simulink model "Transformation_V12"  (R2018a)
settings: Solver=FixedStepDiscrete  StartTime=0.0  StopTime=10.0  RelTol=1e-3
InitFcn:
  | Ts_xadc = 0.1;
values from neighbouring files (symbols this model uses):
  T_25MHz = 1/f_25MHz    (= 4e-08)    [TransformationSkript.m]
  T_mech = 2e-08    [TransformationSkript.m]
libraries: hdlsllib x14, simulink x13, simulink_need_slupdate x1
(part 1 of 3)
settings Model: DataTypeOverride=Off  Creator=trichte  LastModifiedBy=Wendel
settings DataIOCC: LimitDataPoints=on  SaveFormat=Array  SaveOutput=off  SaveTime=off
settings OptimizationCC: BlockReduction=off  ConditionallyExecuteInputs=off  DefaultParameterBehavior=Inlined  LifeSpan=inf
settings DebuggingCC: AlgebraicLoopMsg=error  SolverPrmCheckMsg=warning  SingleTaskRateTransMsg=error  AllowSymbolicDim=off  StrictBusMsg=ErrorOnBusTreatedAsVector  SFUnexpectedBacktrackingDiag=warning  SFNoUnconditionalDefaultTransitionDiag=warning  SFExecutionAtInitializationDiag=none
settings HardwareCC: ProdBitPerPointer=32  ProdBitPerSizeT=32  ProdBitPerPtrDiffT=32  ProdLargestAtomicFloat=None  ProdIntDivRoundTo=Undefined  ProdEndianess=Unspecified  ProdWordSize=32  ProdHWDeviceType=ASIC/FPGA->ASIC/FPGA  ProdEqTarget=off
settings ModelReferenceCC: PropagateSignalLabelsOutOfModel=off
settings CodeAppCC: StateflowObjectComments=on
settings GRTTargetCC: TargetLangStandard=C89/C90 (ANSI)  GeneratePreprocessorConditionals=Disable all
settings ConfigComp: CovMetricSettings=dw  CovHtmlReporting=on  CovSaveCumulativeToWorkspaceVar=on  CovSaveSingleToWorkspaceVar=on  CovExternalEMLEnable=off  CovSFcnEnable=off

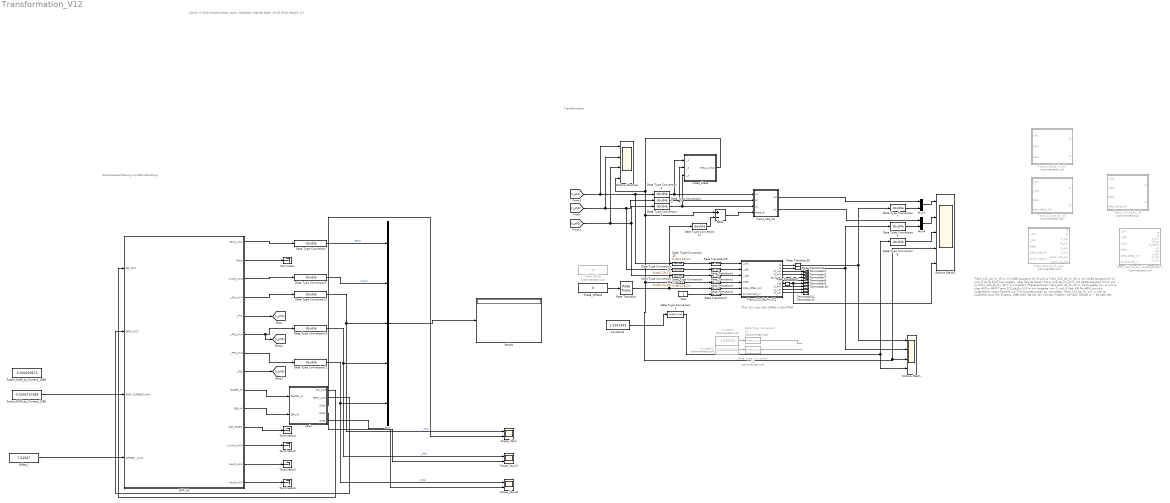
== system Transformation_V12 ==
  note: This V12 runs with 25MHz in the FPGA.
  note: Trans_123_dq_fix_V5 = mit 16Bit Ausgang für id und iq
      | Trans_123_dq_fix_V6 = mit 18 Bit Ausgang für id und iq (iq ist auch hier negativ, aber das ist falsch)
      | Trans_123_dq_fix_V7 = mit 18 Bit Ausgang für id und iq
      | Trans_123_dq_fix_V8 = mit 3 statt 2 Phasenströmen
      | Trans_123_dq_fix_V9 = mit Ausgabe von id und iq über AXI für ARM
      | Trans_123_dq_fix_V10 = mit Ausgabe von i1 und i3 über AXI für ARM und mit zusätzlichem Input-Pipeline um Timingverletzungen zu vermeiden
      | Trans_123_dq_fix_V11 = hier ist zusätzlich auch der Eingang 18Bit breit (da bei der V10 das Problem war das: Sobald iq > 9A geht der Trans-Block nicht mehr richtig...
      | Das liegt an den 16 Bit am Eingang. Sobald ich (wie bei den neunen V11 schon korregiert) 18 Bit am EIngang habe, ist das Problem behoben und der Bereich geht bis bis +/-36 A
      | ...ansonsten is alles wie gehabt. Wegen einheitlichen 18 Bit für alle Größem wird jedoch 18 Bit genutzt!
      | Trans_123_dq_fix_V12 = habe hier nun die dq-Trans von Saidi Said nicht mehr benutzt und bin auf die Verwendung von sinus und cosinus gewechselt.
      | da ich diese bei den VoltageVectors ohnehin benötige. Und hierdurch habe ich auch einen gleichen theta-offset für beide. Außerdem wollte ich alle 3 Ströme nehmen
      | Nach realer Implementierung ist die Genauigkeit von dieser dq-Transformation auch wesentlich genauer (doppelt so gute Bitgenauigkeit)
  note: Stromistwererfassung mit ADC-Wandlung
  note: Transformation
  note: Clarke- & Park-transformation
      |
      | Autor: Sebastian Wendel
      | Date: 26.03.2018
      | Version: 0.1
  Add1 : Sum  Inputs=+-  OutDataTypeStr=Inherit: Same as accumulator
  Constant : Constant  Commented=on  Value=-1.839355
  Constant1 : Constant  Commented=on  Value=0.545410156
  Constant2 : Constant  Value=1.2201433
  DUT_V5 : Subsystem  TreatAsAtomicUnit=on
  Data Type Conversion{,1,3..12} (12 alike) : DataTypeConversion  OutDataTypeStr=double
  Data Type Conversion13 : DataTypeConversion  Commented=on  OutDataTypeStr=fixdt(1,18,11)
  Data Type Conversion14 : DataTypeConversion  Commented=on  OutDataTypeStr=fixdt(1,18,11)
  Data Type Conversion15 : DataTypeConversion  OutDataTypeStr=fixdt(1,18,11)
  Data Type Conversion16 : DataTypeConversion  OutDataTypeStr=fixdt(1,18,11)
  Data Type Conversion17 : DataTypeConversion  OutDataTypeStr=fixdt(1,18,11)
  Data Type Conversion18 : DataTypeConversion  OutDataTypeStr=fixdt(1,24,20)
  Data Type Conversion2 : DataTypeConversion  OutDataTypeStr=fixdt(1,24,20)
  Factor_RAW_to_Current_12Bit : Constant  Value=0.0036747685  OutDataTypeStr=fixdt(0,24,24)
  Factor_RAW_to_Current_16Bit : Constant  Value=0.000229673  OutDataTypeStr=fixdt(0,24,24)
  Mux : Mux  Inputs=5
  Mux3 : Mux  Inputs=2
  Mux4 : Mux  Inputs=2
  Offset_i : Constant  Value=7.52587  OutDataTypeStr=fixdt(0,16,11)
  Rate Transition{,6..7,16} (4 alike) : RateTransition  OutPortSampleTime=T_mech
  Rate Transition{1..5,19} (6 alike) : RateTransition  OutPortSampleTime=T_25MHz
  Scope_Vaux0 : Scope  NumInputPorts=2
  Scope_Vaux8 : Scope  NumInputPorts=2
  Scope_VpVn : Scope  NumInputPorts=2
  Ströme Gleich : Scope  NumInputPorts=4
  Ströme Gleich1 : Scope  NumInputPorts=5
  Ströme Wechsel : Scope  NumInputPorts=4
  Terminator{,1..12} (13 alike) : Terminator
  Test : Constant  OutDataTypeStr=boolean  SampleTime=T_mech
  Theta_Offset : Constant  Commented=on  Value=pi  OutDataTypeStr=fixdt(1,24,20)
  Theta_Offset1 : Constant  Value=0  OutDataTypeStr=fixdt(1,24,20)
  Trans_123_dq : Subsystem
  Trans_123_dq_fix_V11 : Subsystem  Commented=on  TreatAsAtomicUnit=on
  Trans_123_dq_fix_V12 : Subsystem  TreatAsAtomicUnit=on
  Trans_123_dq_fix_V12DoppelteMul : Subsystem  Commented=on  TreatAsAtomicUnit=on
  Trans_123_dq_fix_V3 : Subsystem  Commented=on  TreatAsAtomicUnit=on
  Trans_123_dq_fix_V5 : Subsystem  Commented=on  TreatAsAtomicUnit=on
  Trans_123_dq_fix_V6 : Subsystem  Commented=on  TreatAsAtomicUnit=on
  Values : Display
      settings: Format=hex (Stored Integer)
  meas_theta : Subsystem
  xadc : Subsystem
  wires:
  DUT_V5/1(Temp_AXI4) -> Data Type Conversion/1
  DUT_V5/3(VccInt_AXI4) -> Data Type Conversion1/1
  DUT_V5/4(i_Ph1_AXI4) -> Data Type Conversion3/1
  DUT_V5/7(i_Ph3_AXI4) -> Data Type Conversion11/1
  DUT_V5/6(i_Ph2_AXI4) -> [i_ph2], Data Type Conversion10/1
  Mux/1 -> Values/1
  Data Type Conversion/1 -> Mux/1  "Temp"
  Data Type Conversion3/1 -> Scope_VpVn/1, Mux/3  "i_Ph1"
  Data Type Conversion10/1 -> Scope_Vaux0/1, Mux/4  "i_Ph2"
  Data Type Conversion11/1 -> Scope_Vaux8/1, Mux/5  "i_Ph3"
  Data Type Conversion1/1 -> Mux/2  "VccInt"
  DUT_V5/9(DADDR_IN) -> xadc/1(DADDR_IN)
  DUT_V5/10(DEN_IN) -> xadc/2(DEN_IN)
  xadc/2(DRDY_OUT) -> DUT_V5/2(DRDY_OUT)
  xadc/1(DO_OUT) -> DUT_V5/1(DO_OUT)
  DUT_V5/2(Temp) -> Terminator/1
  DUT_V5/11(ADC_enable) -> Terminator4/1
  Factor_RAW_to_Current_12Bit/1 -> DUT_V5/3(RAW_CURRENT_AXI4)
  Offset_i/1 -> DUT_V5/4(OFFSET_I_AXI4)
  DUT_V5/12(V_VpVn_AXI4) -> Terminator2/1
  DUT_V5/13(Vaux0_AXI4) -> Terminator5/1
  DUT_V5/14(Vaux8_AXI4) -> Terminator6/1
  xadc/3(Sine1) -> Scope_VpVn/2
  xadc/4(Sine2) -> Scope_Vaux0/2
  xadc/5(Sine3) -> Scope_Vaux8/2
  Data Type Conversion2/1 -> Ströme Gleich/4, Data Type Conversion8/1
  Trans_123_dq/1(Ud) -> Mux3/1
  Trans_123_dq/2(Uq) -> Mux4/1
  Mux3/1 -> Ströme Gleich1/1
  Data Type Conversion7/1 -> Mux3/2
  Data Type Conversion6/1 -> Mux4/2
  Mux4/1 -> Ströme Gleich1/2
  Data Type Conversion8/1 -> Ströme Gleich1/3
  meas_theta/1(theta_arctan) -> Ströme Wechsel/4, Ströme Gleich/3, Ströme Gleich1/4, Data Type Conversion18/1, Add1/1
  Data Type Conversion4/1 -> meas_theta/1(I_1), Trans_123_dq/1(L1)
  Data Type Conversion9/1 -> meas_theta/3(I_3), Trans_123_dq/3(L3)
  Data Type Conversion5/1 -> meas_theta/2(I_2), Trans_123_dq/2(L2)
  DUT_V5/5(i_Ph1) -> [i_ph1]
  DUT_V5/8(i_Ph3) -> [i_ph3]
  [i_ph2] -> Ströme Wechsel/2, Data Type Conversion16/1, Data Type Conversion5/1
  Trans_123_dq_fix_V12/1(id) -> Rate Transition16/1
  Trans_123_dq_fix_V12/2(iq) -> Rate Transition6/1
  Data Type Conversion12/1 -> Add1/2
  Add1/1 -> Trans_123_dq/4(theta_el)
  Trans_123_dq_fix_V12/4(iq_AXI) -> Terminator3/1
  Trans_123_dq_fix_V12/3(id_AXI) -> Terminator1/1
  Trans_123_dq_fix_V12/5(dq_Done) -> Terminator7/1
  Trans_123_dq_fix_V12/6(sin) -> Terminator8/1
  [i_ph1] -> Ströme Wechsel/1, Data Type Conversion15/1, Data Type Conversion4/1
  [i_ph3] -> Ströme Wechsel/3, Data Type Conversion17/1, Data Type Conversion9/1
  Data Type Conversion13/1 -> ?
  Data Type Conversion14/1 -> ?
  Rate Transition7/1 -> Ströme Gleich1/5, Terminator9/1
  Test/1 -> Rate Transition5/1
  Trans_123_dq_fix_V12/8(i1_AXI) -> Terminator10/1
  Constant/1 -> Data Type Conversion13/1
  Constant1/1 -> Data Type Conversion14/1
  Constant2/1 -> Data Type Conversion2/1
  Trans_123_dq_fix_V12/9(i2_AXI) -> Terminator11/1
  Trans_123_dq_fix_V12/10(i3_AXI) -> Terminator12/1
  Theta_Offset1/1 -> Rate Transition/1
  Rate Transition19/1 -> Trans_123_dq_fix_V12/1(i_ph1)
  Rate Transition1/1 -> Trans_123_dq_fix_V12/2(i_ph2)
  Rate Transition2/1 -> Trans_123_dq_fix_V12/3(i_ph3)
  Rate Transition3/1 -> Trans_123_dq_fix_V12/4(theta)
  Rate Transition4/1 -> Trans_123_dq_fix_V12/5(theta_offset_AXI)
  Rate Transition5/1 -> Trans_123_dq_fix_V12/6(CurrentValid_in)
  Rate Transition16/1 -> Data Type Conversion7/1, Ströme Gleich/1
  Rate Transition6/1 -> Ströme Gleich/2, Data Type Conversion6/1
  Trans_123_dq_fix_V12/7(cos) -> Rate Transition7/1
  Data Type Conversion15/1 -> Rate Transition19/1
  Data Type Conversion16/1 -> Rate Transition1/1
  Data Type Conversion17/1 -> Rate Transition2/1
  Data Type Conversion18/1 -> Rate Transition3/1
  Rate Transition/1 -> Rate Transition4/1, Data Type Conversion12/1

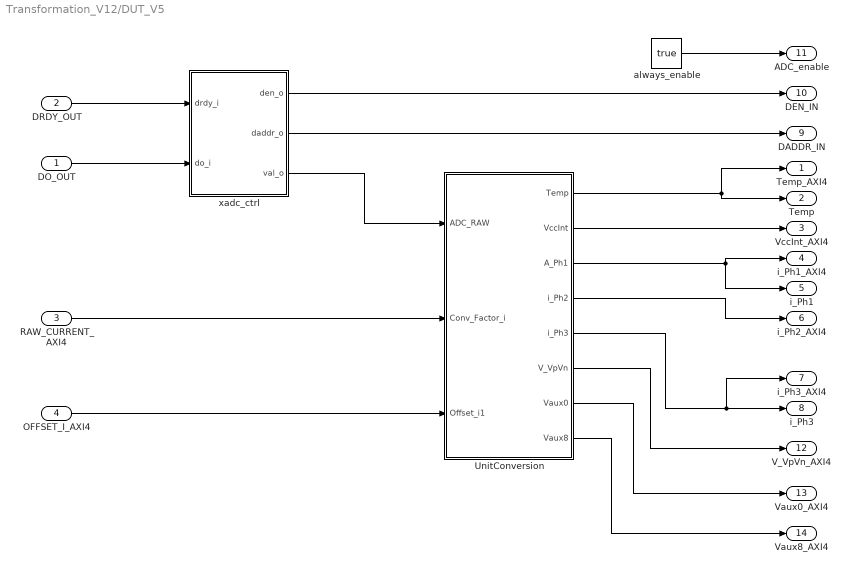
== system Transformation_V12/DUT_V5 ==
  DO_OUT : Inport
  DRDY_OUT : Inport  Port=2
  RAW_CURRENT_AXI4 : Inport  Port=3
  OFFSET_I_AXI4 : Inport  Port=4
  UnitConversion : Subsystem
  always_enable : Constant  Value=true  OutDataTypeStr=boolean
  xadc_ctrl : MATLAB Function  TreatAsAtomicUnit=on
  Temp_AXI4 : Outport
  Temp : Outport  Port=2
  VccInt_AXI4 : Outport  Port=3
  i_Ph1_AXI4 : Outport  Port=4
  i_Ph1 : Outport  Port=5
  i_Ph2_AXI4 : Outport  Port=6
  i_Ph3_AXI4 : Outport  Port=7
  i_Ph3 : Outport  Port=8
  DADDR_IN : Outport  Port=9
  DEN_IN : Outport  Port=10
  ADC_enable : Outport  Port=11
  V_VpVn_AXI4 : Outport  Port=12
  Vaux0_AXI4 : Outport  Port=13
  Vaux8_AXI4 : Outport  Port=14
  wires:
  xadc_ctrl/3(val_o) -> UnitConversion/1(ADC_RAW)
  UnitConversion/5(i_Ph3) -> i_Ph3/1, i_Ph3_AXI4/1
  UnitConversion/3(A_Ph1) -> i_Ph1/1, i_Ph1_AXI4/1
  UnitConversion/4(i_Ph2) -> i_Ph2_AXI4/1
  UnitConversion/2(VccInt) -> VccInt_AXI4/1
  UnitConversion/1(Temp) -> Temp/1, Temp_AXI4/1
  DRDY_OUT/1 -> xadc_ctrl/1(drdy_i)
  DO_OUT/1 -> xadc_ctrl/2(do_i)
  xadc_ctrl/1(den_o) -> DEN_IN/1
  xadc_ctrl/2(daddr_o) -> DADDR_IN/1
  always_enable/1 -> ADC_enable/1
  RAW_CURRENT_AXI4/1 -> UnitConversion/2(Conv_Factor_i)
  UnitConversion/6(V_VpVn) -> V_VpVn_AXI4/1
  OFFSET_I_AXI4/1 -> UnitConversion/3(Offset_i1)
  UnitConversion/7(Vaux0) -> Vaux0_AXI4/1
  UnitConversion/8(Vaux8) -> Vaux8_AXI4/1

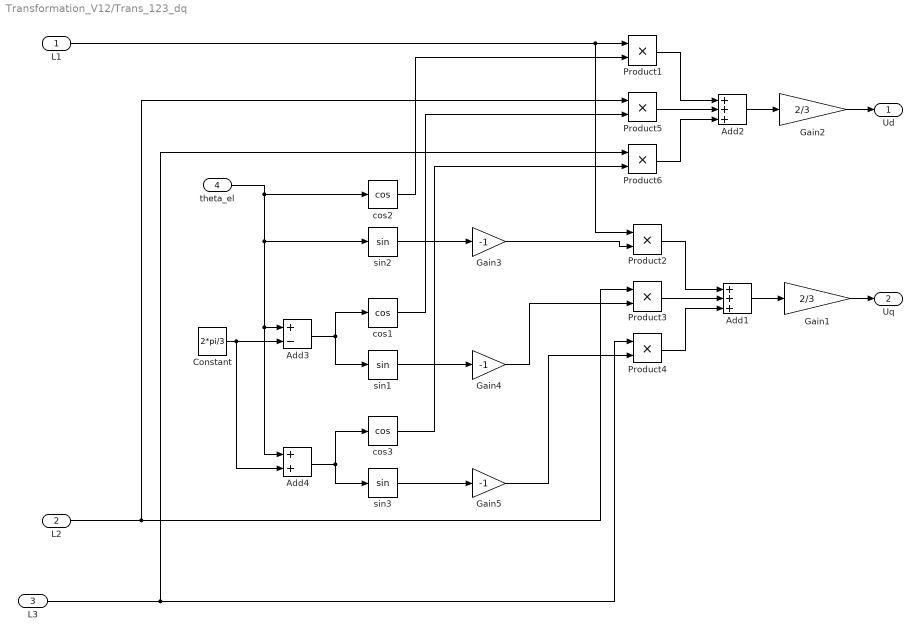
== system Transformation_V12/Trans_123_dq ==
  L1 : Inport
  L2 : Inport  Port=2
  L3 : Inport  Port=3
  theta_el : Inport  Port=4
  Add1 : Sum  Inputs=+++
  Add2 : Sum  Inputs=+++
  Add3 : Sum  Inputs=+-
  Add4 : Sum
  Constant : Constant  Value=2*pi/3  SampleTime=T_mech
  Gain1 : Gain  Gain=2/3
  Gain2 : Gain  Gain=2/3
  Gain3 : Gain  Gain=-1
  Gain4 : Gain  Gain=-1
  Gain5 : Gain  Gain=-1
  Product{1..6} (6 alike) : Product  RndMeth=Zero
  cos1 : Trigonometry  Operator=cos
  cos2 : Trigonometry  Operator=cos
  cos3 : Trigonometry  Operator=cos
  sin1 : Trigonometry
  sin2 : Trigonometry
  sin3 : Trigonometry
  Ud : Outport
  Uq : Outport  Port=2
  wires:
  Gain5/1 -> Product4/2
  Gain4/1 -> Product3/2
  Gain3/1 -> Product2/2
  sin3/1 -> Gain5/1
  sin1/1 -> Gain4/1
  sin2/1 -> Gain3/1
  L3/1 -> Product4/1, Product6/1
  L2/1 -> Product3/1, Product5/1
  L1/1 -> Product2/1, Product1/1
  Gain1/1 -> Uq/1
  Gain2/1 -> Ud/1
  Product6/1 -> Add2/3
  Add2/1 -> Gain2/1
  Product5/1 -> Add2/2
  Product4/1 -> Add1/3
  Add1/1 -> Gain1/1
  Product2/1 -> Add1/1
  Product3/1 -> Add1/2
  theta_el/1 -> cos2/1, Add3/1, Add4/1, sin2/1
  Constant/1 -> Add3/2, Add4/2
  Add3/1 -> cos1/1, sin1/1
  Add4/1 -> cos3/1, sin3/1
  Product1/1 -> Add2/1
  cos3/1 -> Product6/2
  cos1/1 -> Product5/2
  cos2/1 -> Product1/2

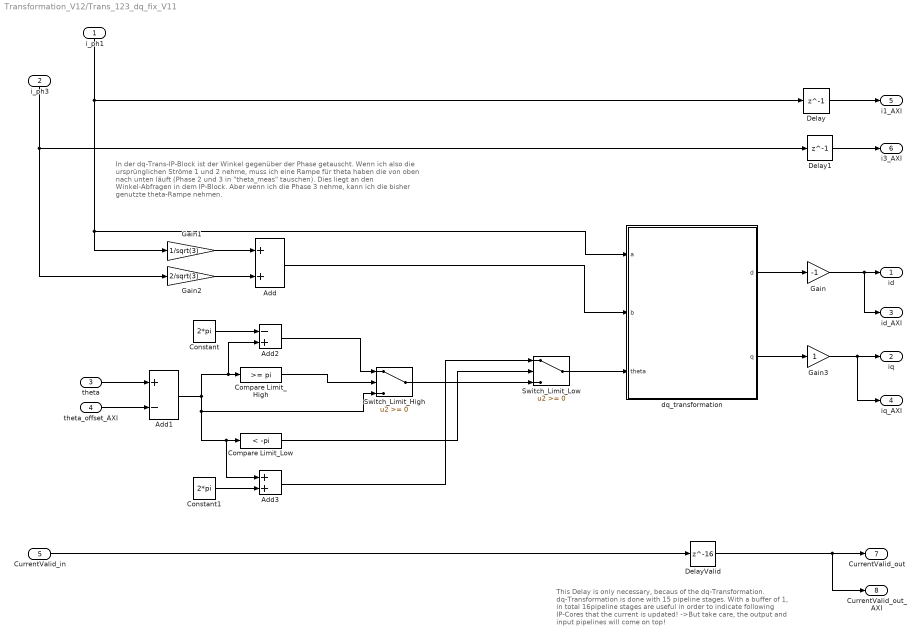
== system Transformation_V12/Trans_123_dq_fix_V11 ==
  note: This Delay is only necessary, becaus of the dq-Transformation.
      | dq-Transformation is done with 15 pipeline stages.
      | With a buffer of 1, in total 16pipeline stages are useful in order to
      |  indicate following IP-Cores that the current is updated!
      | ->But take care, the output and input pipelines will come on top!
  note: In der dq-Trans-IP-Block ist der Winkel gegenüber der Phase getauscht.
      | Wenn ich also die ursprünglichen Ströme 1 und 2 nehme,
      |  muss ich eine Rampe für theta haben die von oben nach unten läuft
      | (Phase 2 und 3 in "theta_meas" tauschen).
      | Dies liegt an den Winkel-Abfragen in dem IP-Block.
      | Aber wenn ich die Phase 3 nehme, kann ich die bisher genutzte theta-Rampe nehmen.
  i_ph1 : Inport
  i_ph3 : Inport  Port=2
  theta : Inport  Port=3
  theta_offset_AXI : Inport  Port=4
  CurrentValid_in : Inport  Port=5
  Add : Sum
  Add1 : Sum  Inputs=+-  OutDataTypeStr=Inherit: Same as accumulator
  Add2 : Sum  Inputs=-+  OutDataTypeStr=Inherit: Same as first input
  Add3 : Sum  OutDataTypeStr=Inherit: Same as first input
  Compare Limit_High : simulink/Logic and Bit Operations/Compare To Constant  relop=>=  const=pi  OutDataTypeStr=boolean
  Compare Limit_Low : simulink/Logic and Bit Operations/Compare To Constant  relop=<  const=-pi  OutDataTypeStr=boolean
  Constant : Constant  Value=2*pi  OutDataTypeStr=fixdt(1,24,20)  SampleTime=-1
  Constant1 : Constant  Value=2*pi  OutDataTypeStr=fixdt(1,24,20)  SampleTime=-1
  Delay : Delay  DelayLength=1
  Delay1 : Delay  DelayLength=1
  DelayValid : Delay  DelayLength=16
  Gain : Gain  Gain=-1  OutDataTypeStr=fixdt(1,18,11)
  Gain1 : Gain  Gain=1/sqrt(3)  OutDataTypeStr=Inherit: Same as input
  Gain2 : Gain  Gain=2/sqrt(3)  OutDataTypeStr=Inherit: Same as input
  Gain3 : Gain  OutDataTypeStr=fixdt(1,18,11)
  Switch_Limit_High : Switch  OutDataTypeStr=fixdt(1,24,20)
  Switch_Limit_Low : Switch  OutDataTypeStr=fixdt(1,24,20)
  dq_transformation : MATLAB Function  TreatAsAtomicUnit=on
  id : Outport
  iq : Outport  Port=2
  id_AXI : Outport  Port=3
  iq_AXI : Outport  Port=4
  i1_AXI : Outport  Port=5
  i3_AXI : Outport  Port=6
  CurrentValid_out : Outport  Port=7
  CurrentValid_out_AXI : Outport  Port=8
  wires:
  Add/1 -> dq_transformation/2(b)
  Gain1/1 -> Add/1
  Gain2/1 -> Add/2
  dq_transformation/2(q) -> Gain3/1
  dq_transformation/1(d) -> Gain/1
  theta/1 -> Add1/1
  Add1/1 -> Switch_Limit_High/3, Add3/1, Compare Limit_Low/1, Add2/2, Compare Limit_High/1
  theta_offset_AXI/1 -> Add1/2
  Switch_Limit_Low/1 -> dq_transformation/3(theta)
  Switch_Limit_High/1 -> Switch_Limit_Low/3
  Compare Limit_High/1 -> Switch_Limit_High/2
  Compare Limit_Low/1 -> Switch_Limit_Low/2
  Constant/1 -> Add2/1
  Add2/1 -> Switch_Limit_High/1
  Constant1/1 -> Add3/2
  Add3/1 -> Switch_Limit_Low/1
  Gain3/1 -> iq_AXI/1, iq/1
  Gain/1 -> id_AXI/1, id/1
  Delay/1 -> i1_AXI/1
  Delay1/1 -> i3_AXI/1
  i_ph3/1 -> Gain2/1, Delay1/1
  i_ph1/1 -> Gain1/1, dq_transformation/1(a), Delay/1
  DelayValid/1 -> CurrentValid_out_AXI/1, CurrentValid_out/1
  CurrentValid_in/1 -> DelayValid/1

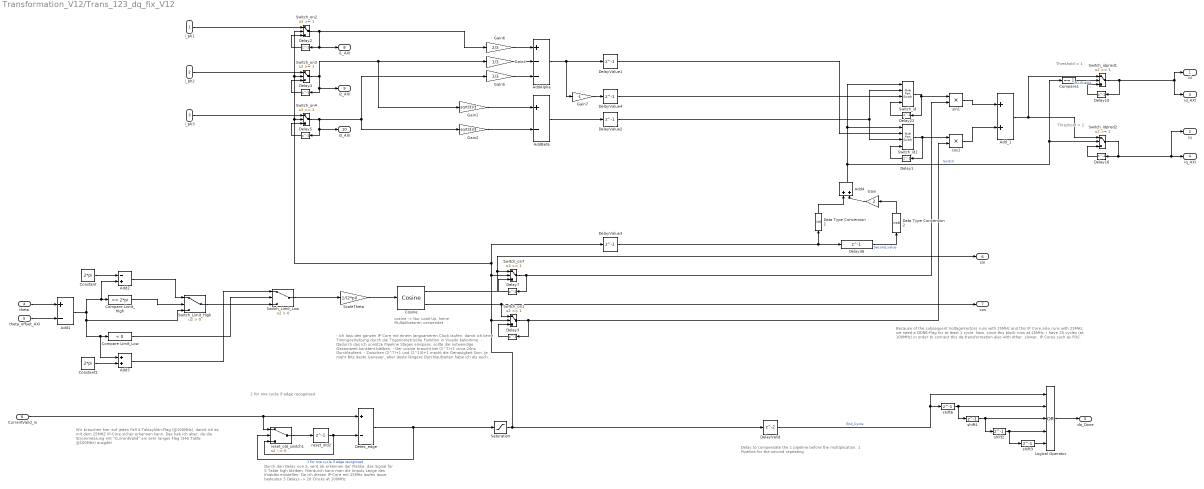
== system Transformation_V12/Trans_123_dq_fix_V12 ==
  note: Delay to compensate the 1 pipeline before the multiplication.
      | 1 Pipeline for the second repeating.
  note: cosine -> Nur Look-Up,
      | keine Multiplikatoren
      | verwendet
  note: - Ich lass den ganzen IP Core mit einem langsameren Clock laufen,
      | damit ich keine Timingverletzung durch die Trigonometrische
      | Funktion in Vivado bekomme.
      | - Dadurch das ich unnütze Pipeline Stages einspare, sollte
      | die notwendige Gesamtzeit konstant bleiben.
      | - Der cosine braucht bei (2^7)+1 circa 24ns Durchlaufzeit.
      | - Zwischen (2^7)+1 und (2^13)+1 macht die Genauigkeit Sinn. Je mehr Bits
      | desto Genauer, aber desto längere Durchlaufzeiten habe ich als auch mehr
      | Ressourcen brauche ich. (Habe mich aktuell für (2^9)+1 entschieden.
  note: Durch den Delay von 5, wird ab erkennen der Flanke,
      |  das Signal für 5 Takte high bleiben.
      | Hierdurch kann man die Impuls Länge des Enables einstellen.
      | Da ich diesen IP-Core mit 25MHz laufen lasse, bedeuten 5 Delays -> 20 Clocks at 100MHz
  note: 1 for one cycle if edge recognized
  note: Wir brauchen hier auf jeden Fall 4 Taktzyklen-Flag (@100MHz),
      | damit ich es mit dem 25MHZ IP-Core sicher erkennen kann. Das hab
      | ich aber, da die Strommessung mit "CurrentValid" ein sehr langes Flag
      | (345 Takte @100MHz) ausgibt!
  note: Because of the subsequent VoltageVectors runs with 25MHz and this
      | IP Core also runs with 25MHz, we need a DONE-Flag for at least 1 cycle.
      | Now, since this block runs at 25MHz, i have 20 cycles (at 100MHz) in order
      | to connect this dq-transformation also with other, slower, IP Cores such as
      | FOC.
  note: Threshold = 1
  note: Threshold = 2
  i_ph1 : Inport
  i_ph2 : Inport  Port=2
  i_ph3 : Inport  Port=3
  theta : Inport  Port=4
  theta_offset_AXI : Inport  Port=5
  CurrentValid_in : Inport  Port=6
  Add1 : Sum  Inputs=+-  OutDataTypeStr=Inherit: Same as accumulator
  Add2 : Sum  Inputs=-+  OutDataTypeStr=Inherit: Same as first input
  Add3 : Sum  OutDataTypeStr=Inherit: Same as first input
  Add4 : Sum  AccumDataTypeStr=int8  OutDataTypeStr=int8  RndMeth=Simplest
  AddAlpha : Sum  Inputs=+--  OutDataTypeStr=Inherit: Same as accumulator
  AddBeta : Sum  Inputs=+-  OutDataTypeStr=Inherit: Same as accumulator
  Add_1 : Sum  OutDataTypeStr=Inherit: Same as accumulator
  Compare Limit_High : simulink/Logic and Bit Operations/Compare To Constant  relop=>=  const=2*pi  OutDataTypeStr=boolean
  Compare Limit_Low : simulink/Logic and Bit Operations/Compare To Constant  relop=<  const=0  OutDataTypeStr=boolean
  Compare1 : simulink/Logic and Bit Operations/Compare To Constant  relop===  const=1  OutDataTypeStr=boolean
  Constant : Constant  Value=2*pi  OutDataTypeStr=fixdt(1,24,20)  SampleTime=T_25MHz
  Constant1 : Constant  Value=2*pi  OutDataTypeStr=fixdt(1,24,20)  SampleTime=T_25MHz
  Cosine : simulink/Lookup Tables/Cosine  Formula=sin(2*pi*u) and cos(2*pi*u)  NumDataPoints=(2^9)+1  OutputWordLength=16  InternalRulePriority=Precision
      settings: SourceProductName=Simulink  SourceProductBaseCode=SL
  Data Type Conversion1 : DataTypeConversion  OutDataTypeStr=int8
  Data Type Conversion2 : DataTypeConversion  OutDataTypeStr=int8
  Delay{1..5,7,10,16,22,36} (10 alike) : Delay  DelayLength=1
  DelayValid : Delay
  DelayValue{1..4} (4 alike) : Delay  DelayLength=1
  Detec_edge : Sum  Inputs=+-  AccumDataTypeStr=int8  OutDataTypeStr=int8
  Gain : Gain  Gain=2  RndMeth=Simplest
  Gain1 : Gain  Gain=sqrt(3)/3  OutDataTypeStr=Inherit: Same as input
  Gain2 : Gain  Gain=sqrt(3)/3  OutDataTypeStr=Inherit: Same as input
  Gain4 : Gain  Gain=1/3  OutDataTypeStr=Inherit: Same as input
  Gain5 : Gain  Gain=1/3  OutDataTypeStr=Inherit: Same as input
  Gain6 : Gain  Gain=2/3  OutDataTypeStr=Inherit: Same as input
  Gain7 : Gain  Gain=-1  OutDataTypeStr=Inherit: Same as input
  Logical Operator : Logic  Operator=OR  Inputs=5  AllPortsSameDT=off  OutDataTypeStr=boolean
  Saturation : Saturate  UpperLimit=1  LowerLimit=0  OutMin=[0]  OutMax=[1]  OutDataTypeStr=fixdt(0,1)
  ScaleTheta : Gain  Gain=1/(2*pi)  OutDataTypeStr=Inherit: Same as input
  Switch_Limit_High : Switch  Criteria=u2 > Threshold  OutDataTypeStr=fixdt(1,24,20)
  Switch_Limit_Low : Switch  Criteria=u2 > Threshold  OutDataTypeStr=fixdt(1,24,20)
  Switch_id : MultiPortSwitch  Inputs=2  DataPortForDefault=Additional data port  DiagnosticForDefault=None  OutDataTypeStr=Inherit: Inherit via back propagation  RndMeth=Simplest
  Switch_id1 : MultiPortSwitch  Inputs=2  DataPortForDefault=Additional data port  DiagnosticForDefault=None  OutDataTypeStr=Inherit: Inherit via back propagation  RndMeth=Simplest
  Switch_idpred1 : Switch  Threshold=1  OutDataTypeStr=Inherit: Inherit via back propagation  RndMeth=Simplest
  Switch_idpred2 : Switch  Threshold=2  OutDataTypeStr=Inherit: Inherit via back propagation  RndMeth=Simplest
  Switch_on1 : Switch  Threshold=1  OutDataTypeStr=fixdt(1,16,14)
  Switch_on2 : Switch  Threshold=1  OutDataTypeStr=Inherit: Inherit via back propagation  RndMeth=Simplest
  Switch_on3 : Switch  Threshold=1  OutDataTypeStr=Inherit: Inherit via back propagation  RndMeth=Simplest
  Switch_on4 : Switch  Threshold=1  OutDataTypeStr=Inherit: Inherit via back propagation  RndMeth=Simplest
  Switch_on7 : Switch  Threshold=1  OutDataTypeStr=fixdt(1,16,14)
  cos1 : Product  RndMeth=Simplest  OutDataTypeStr=Inherit: Same as first input
  reset_old2 : Delay  DelayLength=1
  reset_old_switch1 : Switch  Criteria=u2 ~= 0
  shift{1..3,6} (4 alike) : Delay  DelayLength=1
  sin1 : Product  RndMeth=Simplest  OutDataTypeStr=Inherit: Same as first input
  id : Outport
  iq : Outport  Port=2
  id_AXI : Outport  Port=3
  iq_AXI : Outport  Port=4
  dq_Done : Outport  Port=5
  sin : Outport  Port=6
  cos : Outport  Port=7
  i1_AXI : Outport  Port=8
  i2_AXI : Outport  Port=9
  i3_AXI : Outport  Port=10
  wires:
  Gain1/1 -> AddBeta/1
  Gain2/1 -> AddBeta/2
  theta/1 -> Add1/1
  Add1/1 -> Switch_Limit_High/3, Add3/1, Compare Limit_Low/1, Add2/2, Compare Limit_High/1
  theta_offset_AXI/1 -> Add1/2
  Switch_Limit_High/1 -> Switch_Limit_Low/3
  Compare Limit_High/1 -> Switch_Limit_High/2
  Compare Limit_Low/1 -> Switch_Limit_Low/2
  Constant/1 -> Add2/1
  Add2/1 -> Switch_Limit_High/1
  Constant1/1 -> Add3/2
  Add3/1 -> Switch_Limit_Low/1
  Switch_idpred2/1 -> iq/1, iq_AXI/1, Delay16/1
  Switch_idpred1/1 -> Delay10/1, id/1, id_AXI/1
  Saturation/1 -> DelayValid/1, Switch_on1/2, Switch_on7/2, DelayValue3/1, Switch_on2/2, Switch_on3/2, Switch_on4/2
  Delay3/1 -> Switch_on1/3
  Delay7/1 -> Switch_on7/3
  ScaleTheta/1 -> Cosine/1
  Cosine/2 -> cos/1, Switch_on1/1
  Switch_on7/1 -> Delay7/1, sin1/2
  Cosine/1 -> sin/1, Switch_on7/1
  Switch_on1/1 -> Delay3/1, cos1/2
  Switch_Limit_Low/1 -> ScaleTheta/1
  Gain4/1 -> AddAlpha/2
  Gain5/1 -> AddAlpha/3
  Gain6/1 -> AddAlpha/1
  Detec_edge/1 -> Saturation/1, reset_old_switch1/2  "1 for one cycle if edge recognized"
  reset_old2/1 -> reset_old_switch1/3, Detec_edge/2
  CurrentValid_in/1 -> reset_old_switch1/1, Detec_edge/1
  reset_old_switch1/1 -> reset_old2/1
  Delay2/1 -> Switch_on2/3
  Switch_on2/1 -> Delay2/1, i1_AXI/1, Gain6/1
  i_ph1/1 -> Switch_on2/1
  Switch_on3/1 -> i2_AXI/1, Delay4/1, Gain1/1, Gain4/1
  Delay4/1 -> Switch_on3/3
  i_ph2/1 -> Switch_on3/1
  Switch_on4/1 -> i3_AXI/1, Delay5/1, Gain2/1, Gain5/1
  Delay5/1 -> Switch_on4/3
  i_ph3/1 -> Switch_on4/1
  AddAlpha/1 -> Gain7/1, DelayValue1/1
  AddBeta/1 -> DelayValue2/1
  DelayValid/1 -> shift6/1, Logical Operator/1  "End_Cycle"
  shift6/1 -> Logical Operator/2, shift1/1
  Logical Operator/1 -> dq_Done/1
  Delay10/1 -> Switch_idpred1/3
  Delay16/1 -> Switch_idpred2/3
  Compare1/1 -> Switch_idpred1/2  "id1-Enable"
  Delay22/1 -> Switch_id/4
  Add4/1 -> Switch_idpred2/2, Compare1/1, Switch_id1/1, Switch_id/1  "Switch"
  sin1/1 -> Add_1/1
  cos1/1 -> Add_1/2
  DelayValue1/1 -> Switch_id1/2
  Switch_id/1 -> sin1/1, Delay22/1
  Delay1/1 -> Switch_id1/4
  Switch_id1/1 -> cos1/1, Delay1/1
  DelayValue3/1 -> Data Type Conversion1/1, Delay36/1
  Data Type Conversion1/1 -> Add4/1
  Gain/1 -> Add4/2
  Delay36/1 -> Data Type Conversion2/1  "Second_value"
  Data Type Conversion2/1 -> Gain/1
  DelayValue2/1 -> Switch_id/2, Switch_id1/3
  Add_1/1 -> Switch_idpred1/1, Switch_idpred2/1
  DelayValue4/1 -> Switch_id/3
  Gain7/1 -> DelayValue4/1
  shift1/1 -> Logical Operator/3, shift2/1
  shift2/1 -> shift3/1, Logical Operator/4
  shift3/1 -> Logical Operator/5

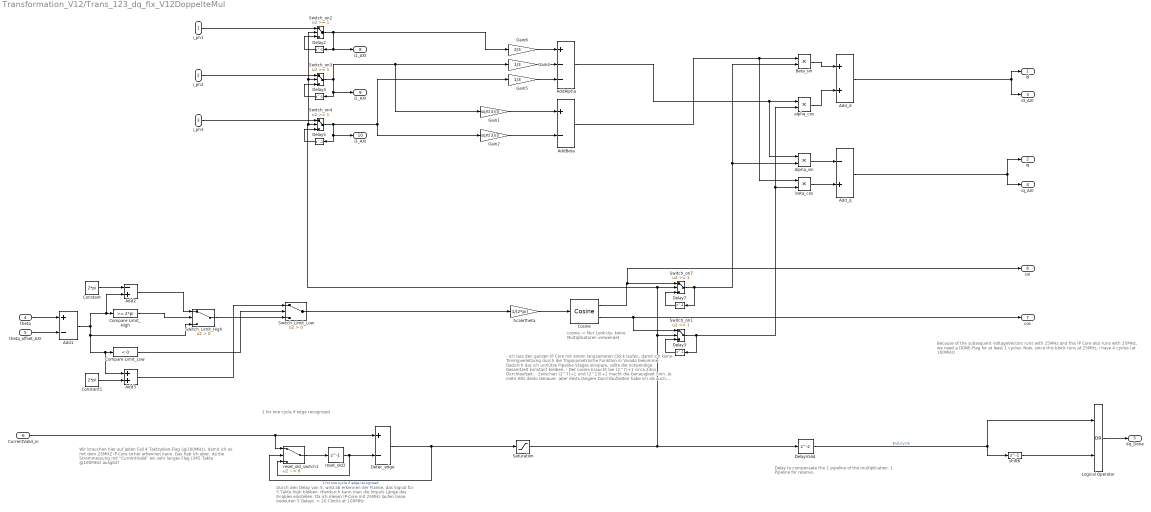
== system Transformation_V12/Trans_123_dq_fix_V12DoppelteMul ==
  note: Delay to compensate the 1 pipeline of the multiplication.
      | 1 Pipeline for reserve.
  note: cosine -> Nur Look-Up,
      | keine Multiplikatoren
      | verwendet
  note: - Ich lass den ganzen IP Core mit einem langsameren Clock laufen,
      | damit ich keine Timingverletzung durch die Trigonometrische
      | Funktion in Vivado bekomme.
      | - Dadurch das ich unnütze Pipeline Stages einspare, sollte
      | die notwendige Gesamtzeit konstant bleiben.
      | - Der cosine braucht bei (2^7)+1 circa 24ns Durchlaufzeit.
      | - Zwischen (2^7)+1 und (2^13)+1 macht die Genauigkeit Sinn. Je mehr Bits
      | desto Genauer, aber desto längere Durchlaufzeiten habe ich als auch mehr
      | Ressourcen brauche ich. (Habe mich aktuell für (2^9)+1 entschieden.
  note: Durch den Delay von 5, wird ab erkennen der Flanke,
      |  das Signal für 5 Takte high bleiben.
      | Hierdurch kann man die Impuls Länge des Enables einstellen.
      | Da ich diesen IP-Core mit 25MHz laufen lasse, bedeuten 5 Delays -> 20 Clocks at 100MHz
  note: 1 for one cycle if edge recognized
  note: Wir brauchen hier auf jeden Fall 4 Taktzyklen-Flag (@100MHz),
      | damit ich es mit dem 25MHZ IP-Core sicher erkennen kann. Das hab
      | ich aber, da die Strommessung mit "CurrentValid" ein sehr langes Flag
      | (345 Takte @100MHz) ausgibt!
  note: Because of the subsequent VoltageVectors runs with 25MHz and this
      | IP Core also runs with 25MHz, we need a DONE-Flag for at least 1 cycles.
      | Now, since this block runs at 25MHz, i have 4 cycles (at 100MHz)
  i_ph1 : Inport
  i_ph2 : Inport  Port=2
  i_ph3 : Inport  Port=3
  theta : Inport  Port=4
  theta_offset_AXI : Inport  Port=5
  CurrentValid_in : Inport  Port=6
  Add1 : Sum  Inputs=+-  OutDataTypeStr=Inherit: Same as accumulator
  Add2 : Sum  Inputs=-+  OutDataTypeStr=Inherit: Same as first input
  Add3 : Sum  OutDataTypeStr=Inherit: Same as first input
  AddAlpha : Sum  Inputs=+--  OutDataTypeStr=Inherit: Same as accumulator  RndMeth=Simplest
  AddBeta : Sum  Inputs=+-  OutDataTypeStr=Inherit: Same as accumulator  RndMeth=Simplest
  Add_d : Sum  OutDataTypeStr=Inherit: Same as accumulator  RndMeth=Simplest
  Add_q : Sum  Inputs=-+  OutDataTypeStr=Inherit: Same as accumulator  RndMeth=Simplest
  Alpha_sin : Product  RndMeth=Simplest  OutDataTypeStr=Inherit: Same as first input
  Beta_sin : Product  RndMeth=Simplest  OutDataTypeStr=Inherit: Same as first input
  Compare Limit_High : simulink/Logic and Bit Operations/Compare To Constant  relop=>=  const=2*pi  OutDataTypeStr=boolean
  Compare Limit_Low : simulink/Logic and Bit Operations/Compare To Constant  relop=<  const=0  OutDataTypeStr=boolean
  Constant : Constant  Value=2*pi  OutDataTypeStr=fixdt(1,24,20)  SampleTime=T_25MHz
  Constant1 : Constant  Value=2*pi  OutDataTypeStr=fixdt(1,24,20)  SampleTime=T_25MHz
  Cosine : simulink/Lookup Tables/Cosine  Formula=sin(2*pi*u) and cos(2*pi*u)  NumDataPoints=(2^9)+1  OutputWordLength=16  InternalRulePriority=Precision
      settings: SourceProductName=Simulink  SourceProductBaseCode=SL
  Delay{2..5,7} (5 alike) : Delay  DelayLength=1
  DelayValid : Delay
  Detec_edge : Sum  Inputs=+-  AccumDataTypeStr=int8  OutDataTypeStr=int8
  Gain1 : Gain  Gain=sqrt(3)/3  OutDataTypeStr=Inherit: Same as input
  Gain2 : Gain  Gain=sqrt(3)/3  OutDataTypeStr=Inherit: Same as input
  Gain4 : Gain  Gain=1/3  OutDataTypeStr=Inherit: Same as input
  Gain5 : Gain  Gain=1/3  OutDataTypeStr=Inherit: Same as input
  Gain6 : Gain  Gain=2/3  OutDataTypeStr=Inherit: Same as input
  Logical Operator : Logic  Operator=OR  AllPortsSameDT=off  OutDataTypeStr=boolean
  Saturation : Saturate  UpperLimit=1  LowerLimit=0  OutMin=[0]  OutMax=[1]  OutDataTypeStr=fixdt(0,1)
  ScaleTheta : Gain  Gain=1/(2*pi)  OutDataTypeStr=Inherit: Same as input
  Switch_Limit_High : Switch  Criteria=u2 > Threshold  OutDataTypeStr=fixdt(1,24,20)
  Switch_Limit_Low : Switch  Criteria=u2 > Threshold  OutDataTypeStr=fixdt(1,24,20)
  Switch_on1 : Switch  Threshold=1  OutDataTypeStr=fixdt(1,16,14)
  Switch_on2 : Switch  Threshold=1  OutDataTypeStr=Inherit: Inherit via back propagation  RndMeth=Simplest
  Switch_on3 : Switch  Threshold=1  OutDataTypeStr=Inherit: Inherit via back propagation  RndMeth=Simplest
  Switch_on4 : Switch  Threshold=1  OutDataTypeStr=Inherit: Inherit via back propagation  RndMeth=Simplest
  Switch_on7 : Switch  Threshold=1  OutDataTypeStr=fixdt(1,16,14)
  alpha_cos : Product  RndMeth=Simplest  OutDataTypeStr=Inherit: Same as first input
  beta_cos : Product  RndMeth=Simplest  OutDataTypeStr=Inherit: Same as first input
  reset_old2 : Delay  DelayLength=1
  reset_old_switch1 : Switch  Criteria=u2 ~= 0
  shift6 : Delay  DelayLength=1
  id : Outport
  iq : Outport  Port=2
  id_AXI : Outport  Port=3
  iq_AXI : Outport  Port=4
  dq_Done : Outport  Port=5
  sin : Outport  Port=6
  cos : Outport  Port=7
  i1_AXI : Outport  Port=8
  i2_AXI : Outport  Port=9
  i3_AXI : Outport  Port=10
  wires:
  Gain1/1 -> AddBeta/1
  Gain2/1 -> AddBeta/2
  theta/1 -> Add1/1
  Add1/1 -> Switch_Limit_High/3, Add3/1, Compare Limit_Low/1, Add2/2, Compare Limit_High/1
  theta_offset_AXI/1 -> Add1/2
  Switch_Limit_High/1 -> Switch_Limit_Low/3
  Compare Limit_High/1 -> Switch_Limit_High/2
  Compare Limit_Low/1 -> Switch_Limit_Low/2
  Constant/1 -> Add2/1
  Add2/1 -> Switch_Limit_High/1
  Constant1/1 -> Add3/2
  Add3/1 -> Switch_Limit_Low/1
  Add_q/1 -> iq/1, iq_AXI/1
  Add_d/1 -> id/1, id_AXI/1
  Saturation/1 -> DelayValid/1, Switch_on1/2, Switch_on2/2, Switch_on3/2, Switch_on4/2, Switch_on7/2
  Delay3/1 -> Switch_on1/3
  Delay7/1 -> Switch_on7/3
  ScaleTheta/1 -> Cosine/1
  Cosine/2 -> Switch_on1/1, cos/1
  Switch_on7/1 -> Delay7/1, Beta_sin/2, Alpha_sin/2
  Cosine/1 -> sin/1, Switch_on7/1
  Switch_on1/1 -> Delay3/1, beta_cos/2, alpha_cos/2
  Switch_Limit_Low/1 -> ScaleTheta/1
  Gain4/1 -> AddAlpha/2
  Gain5/1 -> AddAlpha/3
  Gain6/1 -> AddAlpha/1
  Detec_edge/1 -> Saturation/1, reset_old_switch1/2  "1 for one cycle if edge recognized"
  reset_old2/1 -> reset_old_switch1/3, Detec_edge/2
  CurrentValid_in/1 -> reset_old_switch1/1, Detec_edge/1
  reset_old_switch1/1 -> reset_old2/1
  Delay2/1 -> Switch_on2/3
  Switch_on2/1 -> Delay2/1, i1_AXI/1, Gain6/1
  i_ph1/1 -> Switch_on2/1
  Switch_on3/1 -> i2_AXI/1, Delay4/1, Gain1/1, Gain4/1
  Delay4/1 -> Switch_on3/3
  i_ph2/1 -> Switch_on3/1
  Switch_on4/1 -> i3_AXI/1, Delay5/1, Gain2/1, Gain5/1
  Delay5/1 -> Switch_on4/3
  i_ph3/1 -> Switch_on4/1
  Beta_sin/1 -> Add_d/1
  alpha_cos/1 -> Add_d/2
  AddAlpha/1 -> Alpha_sin/1, alpha_cos/1
  AddBeta/1 -> beta_cos/1, Beta_sin/1
  Alpha_sin/1 -> Add_q/1
  beta_cos/1 -> Add_q/2
  DelayValid/1 -> Logical Operator/1, shift6/1  "End_Cycle"
  shift6/1 -> Logical Operator/2
  Logical Operator/1 -> dq_Done/1

== system Transformation_V12/Trans_123_dq_fix_V3 ==
  i_ph1 : Inport
  i_ph3 : Inport  Port=2
  theta : Inport  Port=3
  Add : Sum
  Gain1 : Gain  Gain=1/sqrt(3)  OutDataTypeStr=Inherit: Same as input
  Gain2 : Gain  Gain=2/sqrt(3)  OutDataTypeStr=Inherit: Same as input
  dq_transformation : MATLAB Function  TreatAsAtomicUnit=on
  id : Outport
  iq : Outport  Port=2
  wires:
  i_ph1/1 -> dq_transformation/1(a), Gain1/1
  Add/1 -> dq_transformation/2(b)
  Gain1/1 -> Add/1
  Gain2/1 -> Add/2
  dq_transformation/2(q) -> iq/1
  dq_transformation/1(d) -> id/1
  i_ph3/1 -> Gain2/1
  theta/1 -> dq_transformation/3(theta)

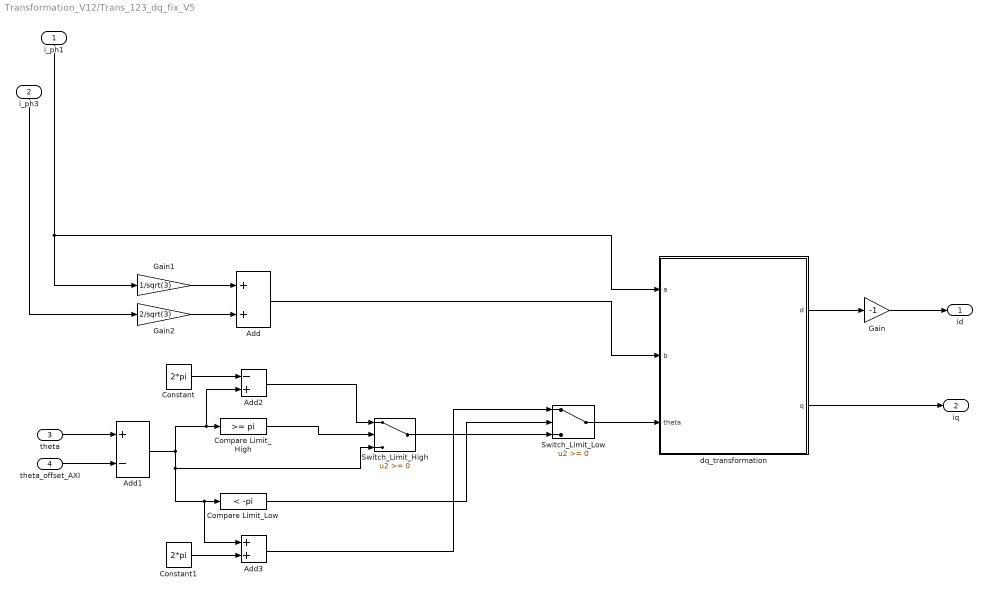
== system Transformation_V12/Trans_123_dq_fix_V5 ==
  i_ph1 : Inport
  i_ph3 : Inport  Port=2
  theta : Inport  Port=3
  theta_offset_AXI : Inport  Port=4
  Add : Sum
  Add1 : Sum  Inputs=+-  OutDataTypeStr=Inherit: Same as accumulator
  Add2 : Sum  Inputs=-+  OutDataTypeStr=Inherit: Same as first input
  Add3 : Sum  OutDataTypeStr=Inherit: Same as first input
  Compare Limit_High : simulink/Logic and Bit Operations/Compare To Constant  relop=>=  const=pi  OutDataTypeStr=boolean
  Compare Limit_Low : simulink/Logic and Bit Operations/Compare To Constant  relop=<  const=-pi  OutDataTypeStr=boolean
  Constant : Constant  Value=2*pi  OutDataTypeStr=fixdt(1,24,20)  SampleTime=-1
  Constant1 : Constant  Value=2*pi  OutDataTypeStr=fixdt(1,24,20)  SampleTime=-1
  Gain : Gain  Gain=-1  OutDataTypeStr=Inherit: Same as input
  Gain1 : Gain  Gain=1/sqrt(3)  OutDataTypeStr=Inherit: Same as input
  Gain2 : Gain  Gain=2/sqrt(3)  OutDataTypeStr=Inherit: Same as input
  Switch_Limit_High : Switch  OutDataTypeStr=fixdt(1,24,20)
  Switch_Limit_Low : Switch  OutDataTypeStr=fixdt(1,24,20)
  dq_transformation : MATLAB Function  TreatAsAtomicUnit=on
  id : Outport
  iq : Outport  Port=2
  wires:
  i_ph1/1 -> dq_transformation/1(a), Gain1/1
  Add/1 -> dq_transformation/2(b)
  Gain1/1 -> Add/1
  Gain2/1 -> Add/2
  dq_transformation/2(q) -> iq/1
  dq_transformation/1(d) -> Gain/1
  i_ph3/1 -> Gain2/1
  theta/1 -> Add1/1
  Add1/1 -> Switch_Limit_High/3, Add3/1, Compare Limit_Low/1, Add2/2, Compare Limit_High/1
  theta_offset_AXI/1 -> Add1/2
  Switch_Limit_Low/1 -> dq_transformation/3(theta)
  Switch_Limit_High/1 -> Switch_Limit_Low/3
  Compare Limit_High/1 -> Switch_Limit_High/2
  Compare Limit_Low/1 -> Switch_Limit_Low/2
  Constant/1 -> Add2/1
  Add2/1 -> Switch_Limit_High/1
  Constant1/1 -> Add3/2
  Add3/1 -> Switch_Limit_Low/1
  Gain/1 -> id/1

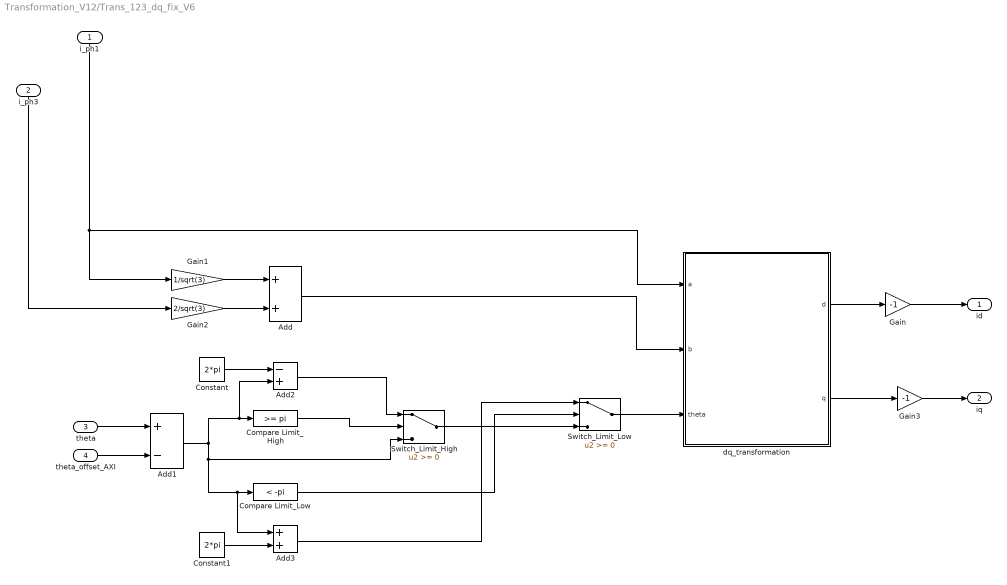
== system Transformation_V12/Trans_123_dq_fix_V6 ==
  i_ph1 : Inport
  i_ph3 : Inport  Port=2
  theta : Inport  Port=3
  theta_offset_AXI : Inport  Port=4
  Add : Sum
  Add1 : Sum  Inputs=+-  OutDataTypeStr=Inherit: Same as accumulator
  Add2 : Sum  Inputs=-+  OutDataTypeStr=Inherit: Same as first input
  Add3 : Sum  OutDataTypeStr=Inherit: Same as first input
  Compare Limit_High : simulink/Logic and Bit Operations/Compare To Constant  relop=>=  const=pi  OutDataTypeStr=boolean
  Compare Limit_Low : simulink/Logic and Bit Operations/Compare To Constant  relop=<  const=-pi  OutDataTypeStr=boolean
  Constant : Constant  Value=2*pi  OutDataTypeStr=fixdt(1,24,20)  SampleTime=-1
  Constant1 : Constant  Value=2*pi  OutDataTypeStr=fixdt(1,24,20)  SampleTime=-1
  Gain : Gain  Gain=-1  OutDataTypeStr=fixdt(1,18,11)
  Gain1 : Gain  Gain=1/sqrt(3)  OutDataTypeStr=Inherit: Same as input
  Gain2 : Gain  Gain=2/sqrt(3)  OutDataTypeStr=Inherit: Same as input
  Gain3 : Gain  Gain=-1  OutDataTypeStr=fixdt(1,18,11)
  Switch_Limit_High : Switch  OutDataTypeStr=fixdt(1,24,20)
  Switch_Limit_Low : Switch  OutDataTypeStr=fixdt(1,24,20)
  dq_transformation : MATLAB Function  TreatAsAtomicUnit=on
  id : Outport
  iq : Outport  Port=2
  wires:
  i_ph1/1 -> dq_transformation/1(a), Gain1/1
  Add/1 -> dq_transformation/2(b)
  Gain1/1 -> Add/1
  Gain2/1 -> Add/2
  dq_transformation/2(q) -> Gain3/1
  dq_transformation/1(d) -> Gain/1
  i_ph3/1 -> Gain2/1
  theta/1 -> Add1/1
  Add1/1 -> Switch_Limit_High/3, Add3/1, Compare Limit_Low/1, Add2/2, Compare Limit_High/1
  theta_offset_AXI/1 -> Add1/2
  Switch_Limit_Low/1 -> dq_transformation/3(theta)
  Switch_Limit_High/1 -> Switch_Limit_Low/3
  Compare Limit_High/1 -> Switch_Limit_High/2
  Compare Limit_Low/1 -> Switch_Limit_Low/2
  Constant/1 -> Add2/1
  Add2/1 -> Switch_Limit_High/1
  Constant1/1 -> Add3/2
  Add3/1 -> Switch_Limit_Low/1
  Gain/1 -> id/1
  Gain3/1 -> iq/1

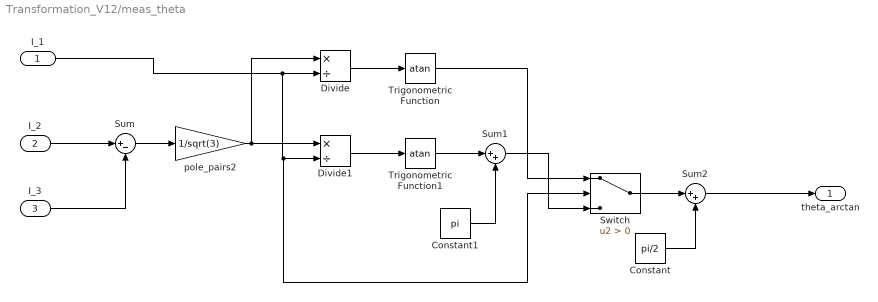
== system Transformation_V12/meas_theta ==
  I_1 : Inport
  I_2 : Inport  Port=2
  I_3 : Inport  Port=3
  Constant : Constant  Value=pi/2
  Constant1 : Constant  Value=pi
  Divide : Product  Inputs=*/
  Divide1 : Product  Inputs=*/
  Sum : Sum  Inputs=|+-
  Sum1 : Sum  Inputs=|++
  Sum2 : Sum  Inputs=|++
  Switch : Switch  Criteria=u2 > Threshold
  Trigonometric Function : Trigonometry  Operator=atan
  Trigonometric Function1 : Trigonometry  Operator=atan
  pole_pairs2 : Gain  Gain=1/sqrt(3)
  theta_arctan : Outport
  wires:
  Divide/1 -> Trigonometric Function/1
  Divide1/1 -> Trigonometric Function1/1
  Trigonometric Function1/1 -> Sum1/1
  pole_pairs2/1 -> Divide/1, Divide1/1
  Sum/1 -> pole_pairs2/1
  I_3/1 -> Sum/2
  I_2/1 -> Sum/1
  I_1/1 -> Switch/2, Divide1/2, Divide/2
  Sum1/1 -> Switch/3
  Trigonometric Function/1 -> Switch/1
  Switch/1 -> Sum2/1
  Constant/1 -> Sum2/2
  Constant1/1 -> Sum1/2
  Sum2/1 -> theta_arctan/1

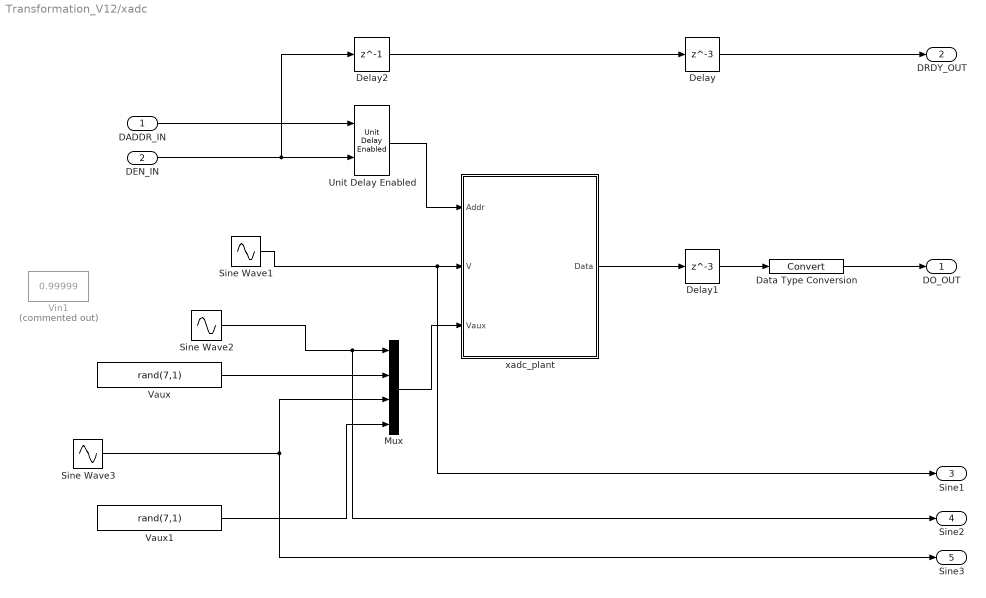
== system Transformation_V12/xadc ==
  DADDR_IN : Inport  OutDataTypeStr=fixdt(0,7,0)
  DEN_IN : Inport  Port=2  OutDataTypeStr=boolean
  Data Type Conversion : DataTypeConversion
  Delay : Delay  DelayLength=3
  Delay1 : Delay  DelayLength=3
  Delay2 : Delay  DelayLength=1
  Mux : Mux
  Sine Wave1 : Sin  Amplitude=0.49  Bias=0.5  Frequency=50  SampleTime=T_mech
  Sine Wave2 : Sin  Amplitude=0.49  Bias=0.5  Frequency=50  Phase=-2*pi/3  SampleTime=T_mech
  Sine Wave3 : Sin  Amplitude=0.49  Bias=0.5  Frequency=50  Phase=2*pi/3  SampleTime=T_mech
  Unit Delay Enabled : simulink_need_slupdate/Unit Delay Enabled  vinit=0.0  tsamp=-1
      settings: SourceProductName=Simulink  SourceProductBaseCode=SL
  Vaux : Constant  Value=rand(7,1)  SampleTime=-1
  Vaux1 : Constant  Value=rand(7,1)  SampleTime=-1
  Vin1 : Constant  Commented=on  Value=0.99999  SampleTime=-1
  xadc_plant : Subsystem
  DO_OUT : Outport  OutDataTypeStr=fixdt(0,16,0)
  DRDY_OUT : Outport  Port=2  OutDataTypeStr=boolean
  Sine1 : Outport  Port=3
  Sine2 : Outport  Port=4
  Sine3 : Outport  Port=5
  wires:
  DEN_IN/1 -> Delay2/1, Unit Delay Enabled/2
  DADDR_IN/1 -> Unit Delay Enabled/1
  Data Type Conversion/1 -> DO_OUT/1
  Delay/1 -> DRDY_OUT/1
  Delay1/1 -> Data Type Conversion/1
  Delay2/1 -> Delay/1
  xadc_plant/1(Data) -> Delay1/1
  Unit Delay Enabled/1 -> xadc_plant/1(Addr)
  Sine Wave1/1 -> Sine1/1, xadc_plant/2(V)
  Vaux/1 -> Mux/2
  Vaux1/1 -> Mux/4
  Sine Wave3/1 -> Mux/3, Sine3/1
  Sine Wave2/1 -> Sine2/1, Mux/1
  Mux/1 -> xadc_plant/3(Vaux)

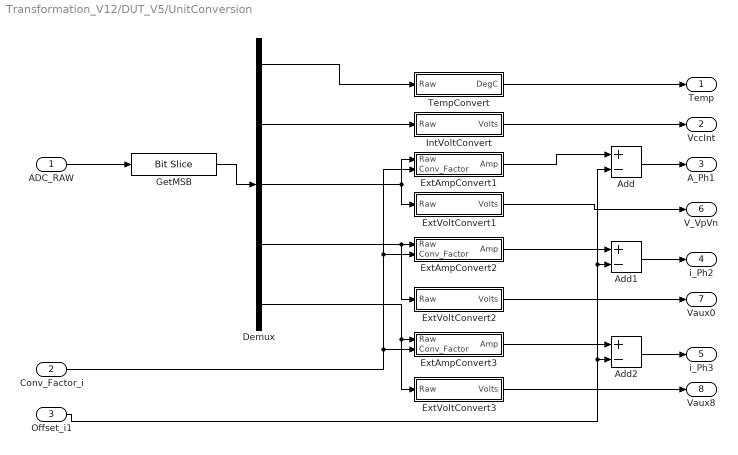
== system Transformation_V12/DUT_V5/UnitConversion ==
  ADC_RAW : Inport
  Conv_Factor_i : Inport  Port=2
  Offset_i1 : Inport  Port=3
  Add : Sum  Inputs=+-  OutDataTypeStr=fixdt(1,16,11)
  Add1 : Sum  Inputs=+-  OutDataTypeStr=fixdt(1,16,11)
  Add2 : Sum  Inputs=+-  OutDataTypeStr=fixdt(1,16,11)
  Demux : Demux  Outputs=5
  ExtAmpConvert1 : Subsystem  TreatAsAtomicUnit=on
  ExtAmpConvert2 : Subsystem  TreatAsAtomicUnit=on
  ExtAmpConvert3 : Subsystem  TreatAsAtomicUnit=on
  ExtVoltConvert1 : Subsystem  TreatAsAtomicUnit=on
  ExtVoltConvert2 : Subsystem  TreatAsAtomicUnit=on
  ExtVoltConvert3 : Subsystem  TreatAsAtomicUnit=on
  GetMSB : hdlsllib/Logic and Bit Operations/Bit Slice  lidx=15  ridx=4
  IntVoltConvert : Subsystem  TreatAsAtomicUnit=on
  TempConvert : Subsystem
  Temp : Outport
  VccInt : Outport  Port=2
  A_Ph1 : Outport  Port=3
  i_Ph2 : Outport  Port=4
  i_Ph3 : Outport  Port=5
  V_VpVn : Outport  Port=6
  Vaux0 : Outport  Port=7
  Vaux8 : Outport  Port=8
  wires:
  ADC_RAW/1 -> GetMSB/1
  GetMSB/1 -> Demux/1
  TempConvert/1(DegC) -> Temp/1
  IntVoltConvert/1(Volts) -> VccInt/1
  ExtAmpConvert1/1(Amp) -> Add/1
  ExtVoltConvert2/1(Volts) -> Vaux0/1
  ExtVoltConvert3/1(Volts) -> Vaux8/1
  Demux/1 -> TempConvert/1(Raw)
  Demux/2 -> IntVoltConvert/1(Raw)
  Demux/3 -> ExtVoltConvert1/1(Raw), ExtAmpConvert1/1(Raw)
  Demux/4 -> ExtVoltConvert2/1(Raw), ExtAmpConvert2/1(Raw)
  Demux/5 -> ExtAmpConvert3/1(Raw), ExtVoltConvert3/1(Raw)
  Conv_Factor_i/1 -> ExtAmpConvert3/2(Conv_Factor), ExtAmpConvert2/2(Conv_Factor), ExtAmpConvert1/2(Conv_Factor)
  ExtVoltConvert1/1(Volts) -> V_VpVn/1
  Add/1 -> A_Ph1/1
  ExtAmpConvert2/1(Amp) -> Add1/1
  Add1/1 -> i_Ph2/1
  ExtAmpConvert3/1(Amp) -> Add2/1
  Add2/1 -> i_Ph3/1
  Offset_i1/1 -> Add2/2, Add/2, Add1/2

== system Transformation_V12/xadc/xadc_plant ==
  Addr : Inport
  V : Inport  Port=2
  Vaux : Inport  Port=3
  AuxChan : Subsystem
  Bit Slice : hdlsllib/Logic and Bit Operations/Bit Slice  lidx=3  ridx=0
  Bit Slice1 : hdlsllib/Logic and Bit Operations/Bit Slice  lidx=4  ridx=4
  IntChan : Subsystem
  Switch : Switch  Criteria=u2 ~= 0
  Data : Outport
  wires:
  Addr/1 -> Bit Slice1/1, Bit Slice/1
  Bit Slice/1 -> IntChan/1(Addr), AuxChan/1(Addr)
  Vaux/1 -> AuxChan/2(Vaux)
  V/1 -> IntChan/2(V)
  Switch/1 -> Data/1
  Bit Slice1/1 -> Switch/2
  IntChan/1(Int_ADC) -> Switch/3
  AuxChan/1(Aux_ADC) -> Switch/1

== system Transformation_V12/DUT_V5/UnitConversion/ExtAmpConvert1 ==
  Raw : Inport
  Conv_Factor : Inport  Port=2
  Product : Product  OutDataTypeStr=fixdt(1,16,11)
  Amp : Outport
  wires:
  Raw/1 -> Product/1
  Product/1 -> Amp/1
  Conv_Factor/1 -> Product/2

== system Transformation_V12/DUT_V5/UnitConversion/ExtAmpConvert2 ==
  Raw : Inport
  Conv_Factor : Inport  Port=2
  Product : Product  OutDataTypeStr=fixdt(1,16,11)
  Amp : Outport
  wires:
  Raw/1 -> Product/1
  Product/1 -> Amp/1
  Conv_Factor/1 -> Product/2

== system Transformation_V12/DUT_V5/UnitConversion/ExtAmpConvert3 ==
  Raw : Inport
  Conv_Factor : Inport  Port=2
  Product : Product  OutDataTypeStr=fixdt(1,16,11)
  Amp : Outport
  wires:
  Raw/1 -> Product/1
  Product/1 -> Amp/1
  Conv_Factor/1 -> Product/2

== system Transformation_V12/DUT_V5/UnitConversion/ExtVoltConvert1 ==
  Raw : Inport
  Gain : Gain  Gain=fi(1/4096)  OutMin=0  OutMax=1  OutDataTypeStr=fixdt(0,16)
  Volts : Outport
  wires:
  Raw/1 -> Gain/1
  Gain/1 -> Volts/1

== system Transformation_V12/DUT_V5/UnitConversion/ExtVoltConvert2 ==
  Raw : Inport
  Gain : Gain  Gain=fi(1/4096)  OutMin=0  OutMax=1  OutDataTypeStr=fixdt(0,16)
  Volts : Outport
  wires:
  Gain/1 -> Volts/1
  Raw/1 -> Gain/1

== system Transformation_V12/DUT_V5/UnitConversion/ExtVoltConvert3 ==
  Raw : Inport
  Gain : Gain  Gain=fi(1/4096)  OutMin=0  OutMax=1  OutDataTypeStr=fixdt(0,16)
  Volts : Outport
  wires:
  Raw/1 -> Gain/1
  Gain/1 -> Volts/1

== system Transformation_V12/DUT_V5/UnitConversion/IntVoltConvert ==
  Raw : Inport
  Gain : Gain  Gain=fi(3/4096)  OutMin=0  OutMax=3  OutDataTypeStr=fixdt(0,16)
  Volts : Outport
  wires:
  Raw/1 -> Gain/1
  Gain/1 -> Volts/1

== system Transformation_V12/DUT_V5/UnitConversion/TempConvert ==
  Raw : Inport
  Add : Sum  Inputs=+-
  Constant : Constant  Value=273.15  OutDataTypeStr=fixdt(0,15)  SampleTime=-1
  Gain : Gain  Gain=fi(503.975/4096)  OutMin=0  OutMax=503.975  OutDataTypeStr=fixdt(0,15)
  DegC : Outport
  wires:
  Gain/1 -> Add/1
  Constant/1 -> Add/2
  Add/1 -> DegC/1
  Raw/1 -> Gain/1

== system Transformation_V12/xadc/xadc_plant/AuxChan ==
  Addr : Inport
  Vaux : Inport  Port=2
  Demux : Demux  Outputs=16
  ExtVoltPlant19 : Subsystem
  Multiport Switch1 : MultiPortSwitch  DataPortOrder=Zero-based contiguous  Inputs=16  DiagnosticForDefault=None  zeroidx=on
  Aux_ADC : Outport
  wires:
  ExtVoltPlant19/1(Raw_ADC) -> Demux/1
  Demux/1 -> Multiport Switch1/2
  Demux/3 -> Multiport Switch1/4
  Demux/2 -> Multiport Switch1/3
  Demux/8 -> Multiport Switch1/9
  Demux/12 -> Multiport Switch1/13
  Demux/6 -> Multiport Switch1/7
  Demux/14 -> Multiport Switch1/15
  Demux/4 -> Multiport Switch1/5
  Demux/10 -> Multiport Switch1/11
  Demux/11 -> Multiport Switch1/12
  Demux/13 -> Multiport Switch1/14
  Demux/5 -> Multiport Switch1/6
  Demux/7 -> Multiport Switch1/8
  Vaux/1 -> ExtVoltPlant19/1(Volts)
  Demux/9 -> Multiport Switch1/10
  Multiport Switch1/1 -> Aux_ADC/1
  Demux/15 -> Multiport Switch1/16
  Addr/1 -> Multiport Switch1/1
  Demux/16 -> Multiport Switch1/17

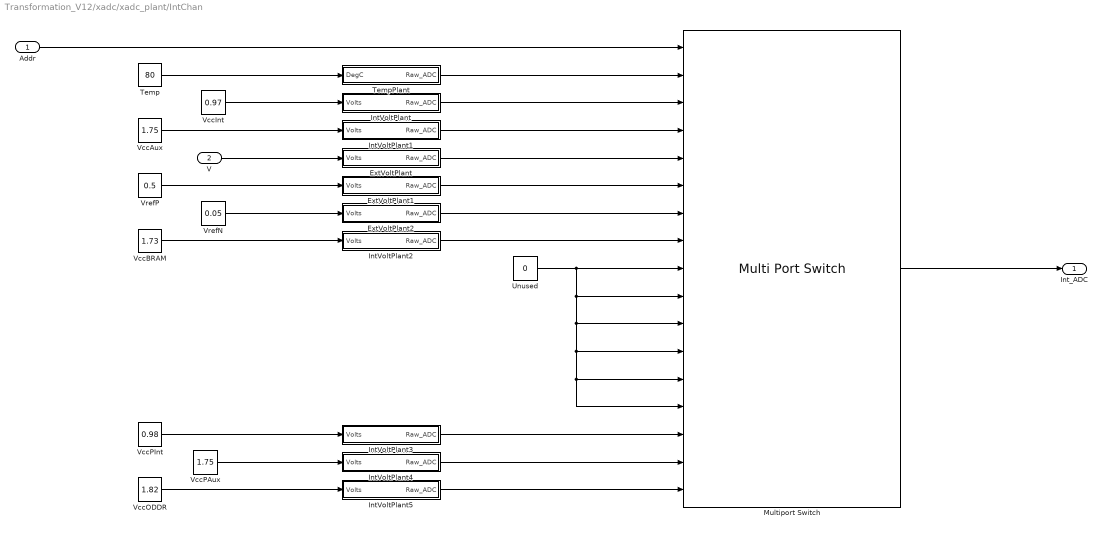
== system Transformation_V12/xadc/xadc_plant/IntChan ==
  Addr : Inport
  V : Inport  Port=2
  ExtVoltPlant : Subsystem
  ExtVoltPlant1 : Subsystem
  ExtVoltPlant2 : Subsystem
  IntVoltPlant : Subsystem
  IntVoltPlant1 : Subsystem
  IntVoltPlant2 : Subsystem
  IntVoltPlant3 : Subsystem
  IntVoltPlant4 : Subsystem
  IntVoltPlant5 : Subsystem
  Multiport Switch : MultiPortSwitch  DataPortOrder=Zero-based contiguous  Inputs=16  DiagnosticForDefault=None  zeroidx=on
  Temp : Constant  Value=80  SampleTime=-1
  TempPlant : Subsystem
  Unused : Constant  Value=0  OutDataTypeStr=Inherit: Inherit via back propagation  SampleTime=-1
  VccAux : Constant  Value=1.75  SampleTime=-1
  VccBRAM : Constant  Value=1.73  SampleTime=-1
  VccInt : Constant  Value=0.97  SampleTime=-1
  VccODDR : Constant  Value=1.82  SampleTime=-1
  VccPAux : Constant  Value=1.75  SampleTime=-1
  VccPInt : Constant  Value=0.98  SampleTime=-1
  VrefN : Constant  Value=0.05  SampleTime=-1
  VrefP : Constant  Value=0.5  SampleTime=-1
  Int_ADC : Outport
  wires:
  IntVoltPlant2/1(Raw_ADC) -> Multiport Switch/8
  VccODDR/1 -> IntVoltPlant5/1(Volts)
  VrefN/1 -> ExtVoltPlant2/1(Volts)
  IntVoltPlant5/1(Raw_ADC) -> Multiport Switch/17
  V/1 -> ExtVoltPlant/1(Volts)
  ExtVoltPlant2/1(Raw_ADC) -> Multiport Switch/7
  TempPlant/1(Raw_ADC) -> Multiport Switch/2
  VccInt/1 -> IntVoltPlant/1(Volts)
  IntVoltPlant4/1(Raw_ADC) -> Multiport Switch/16
  Temp/1 -> TempPlant/1(DegC)
  ExtVoltPlant/1(Raw_ADC) -> Multiport Switch/5
  VccPAux/1 -> IntVoltPlant4/1(Volts)
  VccPInt/1 -> IntVoltPlant3/1(Volts)
  VccAux/1 -> IntVoltPlant1/1(Volts)
  VccBRAM/1 -> IntVoltPlant2/1(Volts)
  IntVoltPlant3/1(Raw_ADC) -> Multiport Switch/15
  Addr/1 -> Multiport Switch/1
  Multiport Switch/1 -> Int_ADC/1
  IntVoltPlant/1(Raw_ADC) -> Multiport Switch/3
  Unused/1 -> Multiport Switch/9, Multiport Switch/14, Multiport Switch/13, Multiport Switch/12, Multiport Switch/11, Multiport Switch/10
  IntVoltPlant1/1(Raw_ADC) -> Multiport Switch/4
  ExtVoltPlant1/1(Raw_ADC) -> Multiport Switch/6
  VrefP/1 -> ExtVoltPlant1/1(Volts)

== system Transformation_V12/xadc/xadc_plant/AuxChan/ExtVoltPlant19 ==
  Volts : Inport
  Bit Concat : hdlsllib/Logic and Bit Operations/Bit Concat  numInputs=2
      settings: SourceProductName=HDL Coder  SourceProductBaseCode=HD
  Data Type Conversion : DataTypeConversion  OutDataTypeStr=fixdt(0,12,0)
  Gain : Gain  Gain=4096
  LSB : Constant  Value=fi(0,0,4,0)  SampleTime=-1
  Raw_ADC : Outport
  wires:
  Bit Concat/1 -> Raw_ADC/1
  LSB/1 -> Bit Concat/2
  Data Type Conversion/1 -> Bit Concat/1
  Volts/1 -> Gain/1
  Gain/1 -> Data Type Conversion/1

== system Transformation_V12/xadc/xadc_plant/IntChan/ExtVoltPlant ==
  Volts : Inport
  Bit Concat : hdlsllib/Logic and Bit Operations/Bit Concat  numInputs=2
      settings: SourceProductName=HDL Coder  SourceProductBaseCode=HD
  Data Type Conversion : DataTypeConversion  OutDataTypeStr=fixdt(0,12,0)
  Gain : Gain  Gain=4096
  LSB : Constant  Value=fi(0,0,4,0)  SampleTime=-1
  Raw_ADC : Outport
  wires:
  Bit Concat/1 -> Raw_ADC/1
  LSB/1 -> Bit Concat/2
  Data Type Conversion/1 -> Bit Concat/1
  Volts/1 -> Gain/1
  Gain/1 -> Data Type Conversion/1

== system Transformation_V12/xadc/xadc_plant/IntChan/ExtVoltPlant1 ==
  Volts : Inport
  Bit Concat : hdlsllib/Logic and Bit Operations/Bit Concat  numInputs=2
      settings: SourceProductName=HDL Coder  SourceProductBaseCode=HD
  Data Type Conversion : DataTypeConversion  OutDataTypeStr=fixdt(0,12,0)
  Gain : Gain  Gain=4096
  LSB : Constant  Value=fi(0,0,4,0)  SampleTime=-1
  Raw_ADC : Outport
  wires:
  Gain/1 -> Data Type Conversion/1
  Volts/1 -> Gain/1
  Data Type Conversion/1 -> Bit Concat/1
  LSB/1 -> Bit Concat/2
  Bit Concat/1 -> Raw_ADC/1

== system Transformation_V12/xadc/xadc_plant/IntChan/ExtVoltPlant2 ==
  Volts : Inport
  Bit Concat : hdlsllib/Logic and Bit Operations/Bit Concat  numInputs=2
      settings: SourceProductName=HDL Coder  SourceProductBaseCode=HD
  Data Type Conversion : DataTypeConversion  OutDataTypeStr=fixdt(0,12,0)
  Gain : Gain  Gain=4096
  LSB : Constant  Value=fi(0,0,4,0)  SampleTime=-1
  Raw_ADC : Outport
  wires:
  Bit Concat/1 -> Raw_ADC/1
  LSB/1 -> Bit Concat/2
  Data Type Conversion/1 -> Bit Concat/1
  Volts/1 -> Gain/1
  Gain/1 -> Data Type Conversion/1

== system Transformation_V12/xadc/xadc_plant/IntChan/IntVoltPlant ==
  Volts : Inport
  Bit Concat : hdlsllib/Logic and Bit Operations/Bit Concat  numInputs=2
      settings: SourceProductName=HDL Coder  SourceProductBaseCode=HD
  Data Type Conversion : DataTypeConversion  OutDataTypeStr=fixdt(0,12,0)
  Gain : Gain  Gain=4096/3
  LSB : Constant  Value=fi(0,0,4,0)  SampleTime=-1
  Raw_ADC : Outport
  wires:
  Gain/1 -> Data Type Conversion/1
  Volts/1 -> Gain/1
  Data Type Conversion/1 -> Bit Concat/1
  LSB/1 -> Bit Concat/2
  Bit Concat/1 -> Raw_ADC/1

== system Transformation_V12/xadc/xadc_plant/IntChan/IntVoltPlant1 ==
  Volts : Inport
  Bit Concat : hdlsllib/Logic and Bit Operations/Bit Concat  numInputs=2
      settings: SourceProductName=HDL Coder  SourceProductBaseCode=HD
  Data Type Conversion : DataTypeConversion  OutDataTypeStr=fixdt(0,12,0)
  Gain : Gain  Gain=4096/3
  LSB : Constant  Value=fi(0,0,4,0)  SampleTime=-1
  Raw_ADC : Outport
  wires:
  Bit Concat/1 -> Raw_ADC/1
  LSB/1 -> Bit Concat/2
  Data Type Conversion/1 -> Bit Concat/1
  Volts/1 -> Gain/1
  Gain/1 -> Data Type Conversion/1

== system Transformation_V12/xadc/xadc_plant/IntChan/IntVoltPlant2 ==
  Volts : Inport
  Bit Concat : hdlsllib/Logic and Bit Operations/Bit Concat  numInputs=2
      settings: SourceProductName=HDL Coder  SourceProductBaseCode=HD
  Data Type Conversion : DataTypeConversion  OutDataTypeStr=fixdt(0,12,0)
  Gain : Gain  Gain=4096/3
  LSB : Constant  Value=fi(0,0,4,0)  SampleTime=-1
  Raw_ADC : Outport
  wires:
  Gain/1 -> Data Type Conversion/1
  Volts/1 -> Gain/1
  Data Type Conversion/1 -> Bit Concat/1
  LSB/1 -> Bit Concat/2
  Bit Concat/1 -> Raw_ADC/1

== system Transformation_V12/xadc/xadc_plant/IntChan/IntVoltPlant3 ==
  Volts : Inport
  Bit Concat : hdlsllib/Logic and Bit Operations/Bit Concat  numInputs=2
      settings: SourceProductName=HDL Coder  SourceProductBaseCode=HD
  Data Type Conversion : DataTypeConversion  OutDataTypeStr=fixdt(0,12,0)
  Gain : Gain  Gain=4096/3
  LSB : Constant  Value=fi(0,0,4,0)  SampleTime=-1
  Raw_ADC : Outport
  wires:
  Bit Concat/1 -> Raw_ADC/1
  LSB/1 -> Bit Concat/2
  Data Type Conversion/1 -> Bit Concat/1
  Volts/1 -> Gain/1
  Gain/1 -> Data Type Conversion/1

== system Transformation_V12/xadc/xadc_plant/IntChan/IntVoltPlant4 ==
  Volts : Inport
  Bit Concat : hdlsllib/Logic and Bit Operations/Bit Concat  numInputs=2
      settings: SourceProductName=HDL Coder  SourceProductBaseCode=HD
  Data Type Conversion : DataTypeConversion  OutDataTypeStr=fixdt(0,12,0)
  Gain : Gain  Gain=4096/3
  LSB : Constant  Value=fi(0,0,4,0)  SampleTime=-1
  Raw_ADC : Outport
  wires:
  Gain/1 -> Data Type Conversion/1
  Volts/1 -> Gain/1
  Data Type Conversion/1 -> Bit Concat/1
  LSB/1 -> Bit Concat/2
  Bit Concat/1 -> Raw_ADC/1
